simulink model "orbit_propagator_matlab2023b"  (R2023b)
settings: Solver=FixedStepAuto  StartTime=0.0  StopTime=207944  FixedStep=sim_step_size  RelTol=1e-6  AbsTol=1e-7
model workspace (MAT data in the model file):
  current_year = 2025
  year = 2013
values from neighbouring files (symbols this model uses):
  alpha_acc = sqrt(0.7)    [HSat_op_setup_merged_maria.m]    (also in init_orbit_analysis_with_drag_loss.m)
  aph = 200*ones(1,7)    [init_orbit_analysis_with_drag_loss.m]
  COM = [0, 0, 0.25+0.3]    [init_orbit_analysis_with_drag_loss.m]
  ext_ENV_muEarth = 3.986005e14    (= 398600500000000)    [GEO_insertion_setup.m]    (also in HSat_op_setup.m; HSat_op_setup_merged_maria.m; init_orbit_analysis_with_drag_loss.m)
  F107 = 300    [init_orbit_analysis_with_drag_loss.m]
  P_solar = 4.56e-6    (= 4.56e-06)    [HSat_op_setup_merged_maria.m]    (also in init_orbit_analysis_with_drag_loss.m)
  perigee_vector_eci = [0, 1, 0]    [init_orbit_analysis_with_drag_loss.m]
  sim_SC_init_MoI_EOR_wet = [ ... (first row only)    [HSat_op_setup.m]    (also in HSat_op_setup_merged_maria.m; init_orbit_analysis_with_drag_loss.m)
  sim_step_size = 10    [init_orbit_analysis_with_drag_loss.m]
  sun_pointing = 1    [init_orbit_analysis_with_drag_loss.m]
  sun_pointing_SA = 0    [HSat_op_setup_merged_maria.m]    (also in init_orbit_analysis_with_drag_loss.m)
  theta = deg2rad(0)    [init_orbit_analysis_with_drag_loss.m]
undefined symbols (not defined in the file or in its folder): attitude, sun_vector_oc
libraries: aerolibutil x37, matrix_library x37, Toolbox x10, sharedtransform x10, aerolibatmos2 x1, simulink x1, simulink_extras x1
(part 1 of 3)
settings Model: Creator=mariahoflund  LastModifiedBy=mariahoflund
settings OptimizationCC: ReuseModelBlockBuffer=off

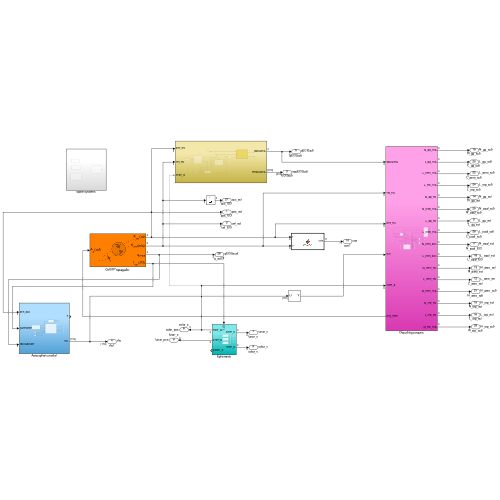
[thumbnail: Simulink's stored preview of the top-level diagram]
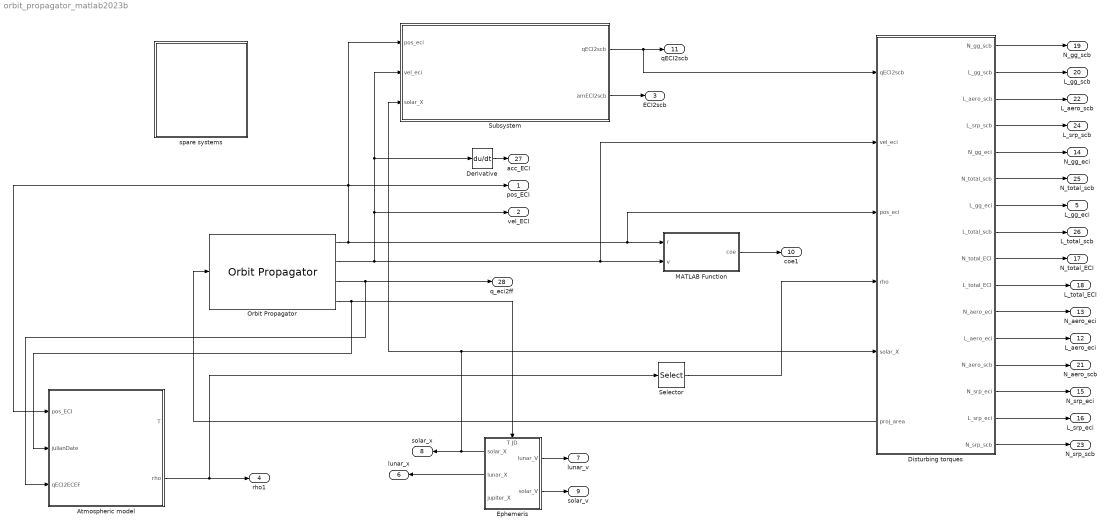
== system orbit_propagator_matlab2023b ==
  Atmospheric model : Subsystem
  Derivative : Derivative
  Disturbing torques : Subsystem
      settings: PortSchema="{\"entries\":[{\"content\":{\"sides\":[{\"content\":{\"connectorIds\":[\"In1\",\"In2\",\"In3\",\"In4\",\"In5\",\"Out17\"]},\"type\":\"ConnectorPlacement.EquallySpacedRectSide\",\"uuid\":\"f7646224-ab06-4eea-96ac-d12bca900cc3\"},{\"content\":{\"connectorIds\":[\"Out1\",\"Out2\",\"Out3\",\"Out4\",\"Out5\",\"Out6\",\"Out7\",\"Out8\",\"Out9\",\"Out10\",\"Out11\",\"Out12\",\"Out13\",\"Out14\",\"Out15\",\"Out16\"],\"side\":\"RIGHT\"},\"type\":\"ConnectorPlacement.EquallySpacedRectSide\",\"uuid\":\"f1692c9b-85c8-425f-b863-5686676bcc52\"},{\"content\":{\"side\":\"TOP\"},\"type\":\"ConnectorPlacement.EquallySpacedRectSide\",\"uuid\":\"99318efc-0d51-43b9-a797-88ad9969849b\"}]},\"type\":\"ConnectorPlacement.EquallySpacedConnector\",\"uuid\":\"1ef90454-3497-43ed-a39d-3078d1204b3e\"}],\"packageUris\":[\"http://schema.mathworks.com/mf0/Connector/R2020b\"],\"version\":\"1.0\"}"
  Ephemeris : Subsystem
      settings: PortSchema="{\"entries\":[{\"content\":{\"sides\":[{\"content\":{\"connectorIds\":[\"Out4\",\"Out5\"]},\"type\":\"ConnectorPlacement.EquallySpacedRectSide\",\"uuid\":\"e633fcf3-0477-4ff0-a81d-4455c68815fb\"},{\"content\":{\"connectorIds\":[\"Out1\",\"Out2\",\"Out3\"],\"side\":\"RIGHT\"},\"type\":\"ConnectorPlacement.EquallySpacedRectSide\",\"uuid\":\"e19e3365-4d80-4524-a5d7-f4214f0f2988\"},{\"content\":{\"connectorIds\":[\"In1\"],\"side\":\"TOP\"},\"type\":\"ConnectorPlacement.EquallySpacedRectSide\",\"uuid\":\"a3adb7cc-79c0-421a-aab6-26119d48c80d\"}]},\"type\":\"ConnectorPlacement.EquallySpacedConnector\",\"uuid\":\"987b98a1-bb11-4f5a-8767-775a43bc92c1\"}],\"packageUris\":[\"http://schema.mathworks.com/mf0/Connector/R2020b\"],\"version\":\"1.0\"}"
  MATLAB Function : MATLAB Function  TreatAsAtomicUnit=on
  Orbit Propagator : OrbitPropagator  propagator=Numerical (high precision)  startDate=2459204.5  mass=mission.Satellite.mass  semiMajorAxis=mission.Satellite.SemiMajorAxis  eccentricity=mission.Satellite.Eccentricity  inclination=mission.Satellite.Inclination  raan=mission.Satellite.RAAN  argPeriapsis=mission.Satellite.ArgOfPeriapsis  trueAnomaly=mission.Satellite.TrueAnomaly  inertialPosition=[3649700.0 3308200.0 -4676600.0]  inertialVelocity=[-2750.8 6666.4 2573.4]  fixedPosition=[-4142689.0 -2676864.7 -4669861.6]  fixedVelocity=[1452.7 -6720.7 2568.1]  customR=3396200  customMu=4.305e13  customJ2=1.0826269e-03  customOmega=4.06125949e-3  shDegree=60  outputTransform=on  useDrag=on  dragCoeff=Cd  dragAreaSrc=Port  dragArea=mission.Satellite.area  includeJupiterGravity=on
  Selector : Selector  InputPortWidth=9  IndexOptions=Index vector (dialog)  Indices=[6]  OutputSizes=1
  Subsystem : Subsystem
  spare systems : Subsystem
  pos_ECI : Outport  SignalName=pos_eci
  vel_ECI : Outport  Port=2  SignalName=vel_eci
  ECI2scb : Outport  Port=3  SignalName=matECI2scb
  rho1 : Outport  Port=4  SignalName=rho
  L_gg_eci : Outport  Port=5  SignalName=L_gg_eci
  lunar_x : Outport  Port=6  SignalName=lunar_pos
  lunar_v : Outport  Port=7  SignalName=lunar_v
  solar_x : Outport  Port=8  SignalName=solar_pos
  solar_v : Outport  Port=9  SignalName=solar_v
  coe1 : Outport  Port=10  SignalName=coe
  qECI2scb : Outport  Port=11  SignalName=qECI2scb
  L_aero_eci : Outport  Port=12  SignalName=L_aero_eci
  N_aero_eci : Outport  Port=13  SignalName=N_aero_eci
  N_gg_eci : Outport  Port=14  SignalName=N_gg_eci
  N_srp_eci : Outport  Port=15  SignalName=N_srp_eci
  L_srp_eci : Outport  Port=16  SignalName=L_srp_eci
  N_total_ECI : Outport  Port=17  SignalName=N_total_eci
  L_total_ECI : Outport  Port=18  SignalName=L_total_eci
  N_gg_scb : Outport  Port=19  SignalName=N_gg_scb
  L_gg_scb : Outport  Port=20  SignalName=L_gg_scb
  N_aero_scb : Outport  Port=21  SignalName=N_aero_scb
  L_aero_scb : Outport  Port=22  SignalName=L_aero_scb
  N_srp_scb : Outport  Port=23  SignalName=N_srp_scb
  L_srp_scb : Outport  Port=24  SignalName=L_srp_scb
  N_total_scb : Outport  Port=25  SignalName=N_total_scb
  L_total_scb : Outport  Port=26  SignalName=L_total_scb
  acc_ECI : Outport  Port=27  SignalName=acc_eci
  q_eci2ff : Outport  Port=28  SignalName=qECI2ecef
  wires:
  Ephemeris/2(lunar_X) -> lunar_x/1
  Orbit Propagator/4 -> Ephemeris/1(T JD), Atmospheric model/2(julianDate)
  MATLAB Function/1(coe) -> coe1/1
  Orbit Propagator/2 -> Subsystem/2(vel_eci), Derivative/1, vel_ECI/1, Disturbing torques/2(vel_eci), MATLAB Function/2(v)
  Ephemeris/4(lunar_V) -> lunar_v/1
  Ephemeris/5(solar_V) -> solar_v/1
  Orbit Propagator/1 -> Atmospheric model/1(pos_ECI), Subsystem/1(pos_eci), pos_ECI/1, MATLAB Function/1(r), Disturbing torques/3(pos_eci)
  Derivative/1 -> acc_ECI/1
  Orbit Propagator/3 -> q_eci2ff/1, Atmospheric model/3(qECI2ECEF)
  Ephemeris/1(solar_X) -> Subsystem/3(solar_X), Disturbing torques/5(solar_X), solar_x/1
  Selector/1 -> Disturbing torques/4(rho)
  Disturbing torques/1(N_gg_scb) -> N_gg_scb/1
  Disturbing torques/2(L_gg_scb) -> L_gg_scb/1
  Disturbing torques/3(L_aero_scb) -> L_aero_scb/1
  Disturbing torques/4(L_srp_scb) -> L_srp_scb/1
  Disturbing torques/5(N_gg_eci) -> N_gg_eci/1
  Disturbing torques/6(N_total_scb) -> N_total_scb/1
  Disturbing torques/7(L_gg_eci) -> L_gg_eci/1
  Disturbing torques/8(L_total_scb) -> L_total_scb/1
  Disturbing torques/9(N_total_ECI) -> N_total_ECI/1
  Disturbing torques/17(proj_area) -> Orbit Propagator/1
  Disturbing torques/10(L_total_ECI) -> L_total_ECI/1
  Disturbing torques/11(N_aero_eci) -> N_aero_eci/1
  Disturbing torques/12(L_aero_eci) -> L_aero_eci/1
  Disturbing torques/13(N_aero_scb) -> N_aero_scb/1
  Disturbing torques/14(N_srp_eci) -> N_srp_eci/1
  Disturbing torques/15(L_srp_eci) -> L_srp_eci/1
  Disturbing torques/16(N_srp_scb) -> N_srp_scb/1
  Atmospheric model/2(rho) -> rho1/1, Selector/1
  Subsystem/1(qECI2scb) -> Disturbing torques/1(qECI2scb), qECI2scb/1
  Subsystem/2(amECI2scb) -> ECI2scb/1

== system orbit_propagator_matlab2023b/Atmospheric model ==
  pos_ECI : Inport
  julianDate : Inport  Port=2
  qECI2ECEF : Inport  Port=3
  F107 : Constant  Value=F107
  F107a : Constant  Value=F107
  MATLAB Function1 : MATLAB Function  TreatAsAtomicUnit=on
  NRLMSISE-00 Atmosphere Model : aerolibatmos2/NRLMSISE-00 Atmosphere Model  units=Metric (MKS)  lst_input=off  flux_ap_input=on  flags_input=Internal  flags=ones(1,23)  oxygen_in=off  action=Warning
  aph : Constant  Value=aph
  pos_eci to lla : Subsystem
  T : Outport
  rho : Outport  Port=2
  wires:
  NRLMSISE-00 Atmosphere Model/2 -> rho/1
  qECI2ECEF/1 -> pos_eci to lla/2(qECI2ECEF)
  julianDate/1 -> MATLAB Function1/1(julianDate)
  F107/1 -> NRLMSISE-00 Atmosphere Model/6
  NRLMSISE-00 Atmosphere Model/1 -> T/1
  MATLAB Function1/1(yr) -> NRLMSISE-00 Atmosphere Model/2
  pos_ECI/1 -> pos_eci to lla/1(pos_ECI)
  aph/1 -> NRLMSISE-00 Atmosphere Model/7
  MATLAB Function1/2(dayOfYear) -> NRLMSISE-00 Atmosphere Model/3
  pos_eci to lla/1(Out1) -> NRLMSISE-00 Atmosphere Model/1  "lat,long,alt"
  F107a/1 -> NRLMSISE-00 Atmosphere Model/5
  MATLAB Function1/3(timeUTSeconds) -> NRLMSISE-00 Atmosphere Model/4

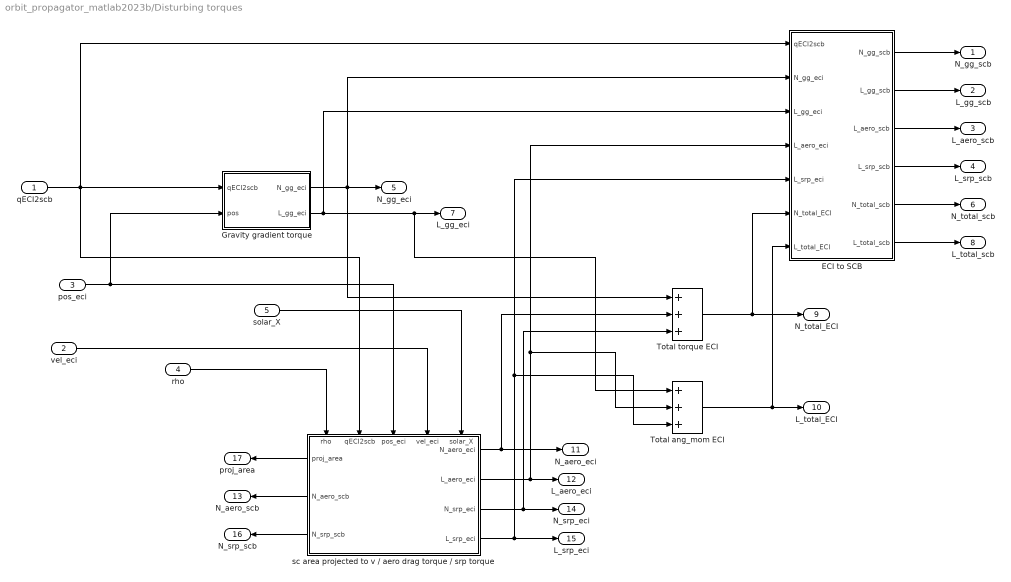
== system orbit_propagator_matlab2023b/Disturbing torques ==
  qECI2scb : Inport
  vel_eci : Inport  Port=2
  pos_eci : Inport  Port=3
  rho : Inport  Port=4
  solar_X : Inport  Port=5
  ECI to SCB : Subsystem
  Gravity gradient torque : Subsystem
  Total ang_mom ECI : Sum  Inputs=+++
  Total torque ECI : Sum  Inputs=+++
  sc area projected to v / aero drag torque / srp torque : Subsystem
      settings: PortSchema="{\"entries\":[{\"content\":{\"sides\":[{\"content\":{\"connectorIds\":[\"Out5\",\"Out6\",\"Out7\"]},\"type\":\"ConnectorPlacement.EquallySpacedRectSide\",\"uuid\":\"2286bbd5-74fd-4e7a-af53-1dba63e33399\"},{\"content\":{\"connectorIds\":[\"Out1\",\"Out2\",\"Out3\",\"Out4\"],\"side\":\"RIGHT\"},\"type\":\"ConnectorPlacement.EquallySpacedRectSide\",\"uuid\":\"14ee861f-d330-4e3d-9d37-eadf89803ba2\"},{\"content\":{\"connectorIds\":[\"In1\",\"In2\",\"In3\",\"In4\",\"In5\"],\"side\":\"TOP\"},\"type\":\"ConnectorPlacement.EquallySpacedRectSide\",\"uuid\":\"a82f7821-7262-41d9-9ef8-416bfb7d6f77\"}]},\"type\":\"ConnectorPlacement.EquallySpacedConnector\",\"uuid\":\"26570817-76bd-4bb8-9b49-7b0dee7f17a2\"}],\"packageUris\":[\"http://schema.mathworks.com/mf0/Connector/R2020b\"],\"version\":\"1.0\"}"
  N_gg_scb : Outport
  L_gg_scb : Outport  Port=2
  L_aero_scb : Outport  Port=3
  L_srp_scb : Outport  Port=4
  N_gg_eci : Outport  Port=5
  N_total_scb : Outport  Port=6
  L_gg_eci : Outport  Port=7
  L_total_scb : Outport  Port=8
  N_total_ECI : Outport  Port=9
  L_total_ECI : Outport  Port=10
  N_aero_eci : Outport  Port=11
  L_aero_eci : Outport  Port=12
  N_aero_scb : Outport  Port=13
  N_srp_eci : Outport  Port=14
  L_srp_eci : Outport  Port=15
  N_srp_scb : Outport  Port=16
  proj_area : Outport  Port=17
  wires:
  pos_eci/1 -> Gravity gradient torque/2(pos), sc area projected to v / aero drag torque / srp torque/3(pos_eci)
  sc area projected to v / aero drag torque / srp torque/5(proj_area) -> proj_area/1
  Gravity gradient torque/2(L_gg_eci) -> L_gg_eci/1, Total ang_mom ECI/1, ECI to SCB/3(L_gg_eci)
  sc area projected to v / aero drag torque / srp torque/4(L_srp_eci) -> ECI to SCB/5(L_srp_eci), Total ang_mom ECI/3, L_srp_eci/1
  rho/1 -> sc area projected to v / aero drag torque / srp torque/1(rho)
  ECI to SCB/4(L_srp_scb) -> L_srp_scb/1
  ECI to SCB/5(N_total_scb) -> N_total_scb/1
  solar_X/1 -> sc area projected to v / aero drag torque / srp torque/5(solar_X)
  ECI to SCB/3(L_aero_scb) -> L_aero_scb/1
  sc area projected to v / aero drag torque / srp torque/3(N_srp_eci) -> Total torque ECI/3, N_srp_eci/1
  Total torque ECI/1 -> ECI to SCB/6(N_total_ECI), N_total_ECI/1
  ECI to SCB/6(L_total_scb) -> L_total_scb/1
  ECI to SCB/2(L_gg_scb) -> L_gg_scb/1
  sc area projected to v / aero drag torque / srp torque/1(N_aero_eci) -> Total torque ECI/2, N_aero_eci/1
  ECI to SCB/1(N_gg_scb) -> N_gg_scb/1
  Total ang_mom ECI/1 -> ECI to SCB/7(L_total_ECI), L_total_ECI/1
  qECI2scb/1 -> ECI to SCB/1(qECI2scb), sc area projected to v / aero drag torque / srp torque/2(qECI2scb), Gravity gradient torque/1(qECI2scb)
  sc area projected to v / aero drag torque / srp torque/7(N_srp_scb) -> N_srp_scb/1
  Gravity gradient torque/1(N_gg_eci) -> Total torque ECI/1, N_gg_eci/1, ECI to SCB/2(N_gg_eci)
  sc area projected to v / aero drag torque / srp torque/6(N_aero_scb) -> N_aero_scb/1
  vel_eci/1 -> sc area projected to v / aero drag torque / srp torque/4(vel_eci)
  sc area projected to v / aero drag torque / srp torque/2(L_aero_eci) -> ECI to SCB/4(L_aero_eci), Total ang_mom ECI/2, L_aero_eci/1

== system orbit_propagator_matlab2023b/Ephemeris ==
  T JD : Inport
  Gain{,1..3} (4 alike) : Gain  Gain=1000
  Jupiter Ephemeris : PlanetaryEphem  target=Jupiter
  Lunar Ephemeris : PlanetaryEphem
  Solar Ephemeris : PlanetaryEphem  target=Sun
  km to m : Gain  Gain=1000
  km to m1 : Gain  Gain=1000
  solar_X : Outport
  lunar_X : Outport  Port=2
  jupiter_X : Outport  Port=3
  lunar_V : Outport  Port=4
  solar_V : Outport  Port=5
  wires:
  T JD/1 -> Lunar Ephemeris/1, Jupiter Ephemeris/1, Solar Ephemeris/1
  Lunar Ephemeris/2 -> Gain1/1
  Solar Ephemeris/1 -> Gain2/1
  Solar Ephemeris/2 -> km to m/1
  Lunar Ephemeris/1 -> Gain/1
  Gain/1 -> lunar_X/1
  Gain1/1 -> lunar_V/1
  Gain2/1 -> solar_X/1
  km to m/1 -> solar_V/1
  Jupiter Ephemeris/2 -> km to m1/1
  Gain3/1 -> jupiter_X/1
  km to m1/1 -> ?
  Jupiter Ephemeris/1 -> Gain3/1

== system orbit_propagator_matlab2023b/Subsystem ==
  pos_eci : Inport
  vel_eci : Inport  Port=2
  solar_X : Inport  Port=3
  Attitude : Subsystem  Variant=on  VariantControlMode=label  VariantControl=Choice  LabelModeActiveChoice=nadir  PropagateVariantConditions=on
  Constant : Constant  Value=sun_pointing
  Merge : Merge
  Switch Case : SwitchCase
  sun pointing in orbit plane : Subsystem  TreatAsAtomicUnit=on
  sun pointing out of plane : Subsystem  TreatAsAtomicUnit=on
  qECI2scb : Outport
  amECI2scb : Outport  Port=2
  wires:
  Attitude/1(qECI2scb) -> qECI2scb/1
  vel_eci/1 -> sun pointing in orbit plane/2(vel_eci), Attitude/2(velECI)
  Attitude/2(amECI2scb) -> amECI2scb/1
  pos_eci/1 -> sun pointing in orbit plane/3(pos_eci), Attitude/1(posECI)
  Switch Case/2 -> sun pointing out of plane/Action
  Switch Case/1 -> sun pointing in orbit plane/Action
  solar_X/1 -> sun pointing in orbit plane/1(solar_X), sun pointing out of plane/1(solar_X)
  sun pointing in orbit plane/1(Out1) -> Merge/1
  sun pointing out of plane/1(Out1) -> Merge/2
  Merge/1 -> Attitude/3(solar_X)
  Constant/1 -> Switch Case/1

== system orbit_propagator_matlab2023b/spare systems ==
  LST calculation : Subsystem  Commented=on
  Subsystem : Subsystem  Commented=on
  create custom sun vector : Subsystem  Commented=on
      settings: PortSchema="{\"entries\":[{\"content\":{\"sides\":[{\"content\":{},\"type\":\"ConnectorPlacement.EquallySpacedRectSide\",\"uuid\":\"5755fe33-27e5-4fac-b1a9-828212356ffb\"},{\"content\":{\"connectorIds\":[\"Out1\"],\"side\":\"RIGHT\"},\"type\":\"ConnectorPlacement.EquallySpacedRectSide\",\"uuid\":\"342e2dfb-ebd3-43c9-8218-dffda7908936\"},{\"content\":{\"connectorIds\":[\"In1\",\"In2\"],\"side\":\"TOP\"},\"type\":\"ConnectorPlacement.EquallySpacedRectSide\",\"uuid\":\"c86662bf-fbb1-4b53-aebd-7f62bd217376\"}]},\"type\":\"ConnectorPlacement.EquallySpacedConnector\",\"uuid\":\"2e470c5a-53cc-4a23-914f-bd86fdc85ade\"}],\"packageUris\":[\"http://schema.mathworks.com/mf0/Connector/R2020b\"],\"version\":\"1.0\"}"
  sun_angle_slo : Subsystem  Commented=on
      settings: PortSchema="{\"entries\":[{\"content\":{\"sides\":[{\"content\":{\"connectorIds\":[\"In1\",\"In2\"]},\"type\":\"ConnectorPlacement.EquallySpacedRectSide\",\"uuid\":\"2286bbd5-74fd-4e7a-af53-1dba63e33399\"},{\"content\":{\"side\":\"RIGHT\"},\"type\":\"ConnectorPlacement.EquallySpacedRectSide\",\"uuid\":\"14ee861f-d330-4e3d-9d37-eadf89803ba2\"},{\"content\":{\"side\":\"TOP\"},\"type\":\"ConnectorPlacement.EquallySpacedRectSide\",\"uuid\":\"a82f7821-7262-41d9-9ef8-416bfb7d6f77\"},{\"content\":{\"connectorIds\":[\"Out1\"],\"side\":\"BOTTOM\"},\"type\":\"ConnectorPlacement.EquallySpacedRectSide\",\"uuid\":\"582a2bf6-c053-407d-b600-dfbf3f97abd6\"}]},\"type\":\"ConnectorPlacement.EquallySpacedConnector\",\"uuid\":\"26570817-76bd-4bb8-9b49-7b0dee7f17a2\"}],\"packageUris\":[\"http://schema.mathworks.com/mf0/Connector/R2020b\"],\"version\":\"1.0\"}"

== system orbit_propagator_matlab2023b/Atmospheric model/pos_eci to lla ==
  pos_ECI : Inport
  qECI2ECEF : Inport  Port=2
  ECEF Position to LLA : ECEF2LLA
  Mux : Mux  Inputs=2
  Quaternion Rotation : aerolibutil/Quaternion Rotation
  Out1 : Outport
  wires:
  pos_ECI/1 -> Quaternion Rotation/2
  qECI2ECEF/1 -> Quaternion Rotation/1
  Quaternion Rotation/1 -> ECEF Position to LLA/1
  ECEF Position to LLA/1 -> Mux/1
  ECEF Position to LLA/2 -> Mux/2
  Mux/1 -> Out1/1

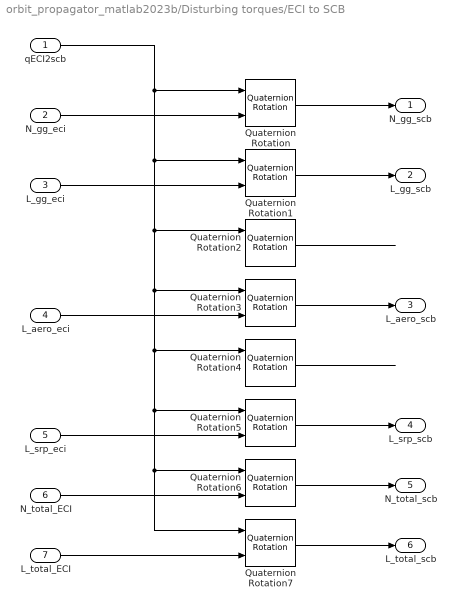
== system orbit_propagator_matlab2023b/Disturbing torques/ECI to SCB ==
  qECI2scb : Inport
  N_gg_eci : Inport  Port=2
  L_gg_eci : Inport  Port=3
  L_aero_eci : Inport  Port=4
  L_srp_eci : Inport  Port=5
  N_total_ECI : Inport  Port=6
  L_total_ECI : Inport  Port=7
  Quaternion Rotation{,1..7} (8 alike) : aerolibutil/Quaternion Rotation
  N_gg_scb : Outport
  L_gg_scb : Outport  Port=2
  L_aero_scb : Outport  Port=3
  L_srp_scb : Outport  Port=4
  N_total_scb : Outport  Port=5
  L_total_scb : Outport  Port=6
  wires:
  qECI2scb/1 -> Quaternion Rotation1/1, Quaternion Rotation2/1, Quaternion Rotation3/1, Quaternion Rotation4/1, Quaternion Rotation7/1, Quaternion Rotation6/1, Quaternion Rotation5/1, Quaternion Rotation/1
  N_gg_eci/1 -> Quaternion Rotation/2
  Quaternion Rotation/1 -> N_gg_scb/1
  Quaternion Rotation1/1 -> L_gg_scb/1
  L_gg_eci/1 -> Quaternion Rotation1/2
  Quaternion Rotation2/1 -> ?
  ? -> Quaternion Rotation2/2
  Quaternion Rotation3/1 -> L_aero_scb/1
  L_aero_eci/1 -> Quaternion Rotation3/2
  Quaternion Rotation4/1 -> ?
  ? -> Quaternion Rotation4/2
  Quaternion Rotation5/1 -> L_srp_scb/1
  L_srp_eci/1 -> Quaternion Rotation5/2
  Quaternion Rotation6/1 -> N_total_scb/1
  Quaternion Rotation7/1 -> L_total_scb/1
  L_total_ECI/1 -> Quaternion Rotation7/2
  N_total_ECI/1 -> Quaternion Rotation6/2

== system orbit_propagator_matlab2023b/Disturbing torques/Gravity gradient torque ==
  qECI2scb : Inport
  pos : Inport  Port=2
  Constant4 : Constant  Value=sim_SC_init_MoI_EOR_wet
  Constant5 : Constant  Value=-5
  Constant6 : Constant  Value=3
  Constant7 : Constant  Value=ext_ENV_muEarth
  Cross Product1 : matrix_library/Cross Product
  Dot Product1 : DotProduct  OutDataTypeStr=Inherit: Inherit via internal rule
  Integrator : Integrator
  Math Function1 : Math  Operator=pow
  Product1 : Product  Inputs=4
  Product2 : Product  Multiplication=Matrix(*)
  Quaternion Inverse : aerolibutil/Quaternion Inverse
  Quaternion Rotation : aerolibutil/Quaternion Rotation
  Quaternion Rotation1 : aerolibutil/Quaternion Rotation
  Sqrt1 : Sqrt
  N_gg_eci : Outport
  L_gg_eci : Outport  Port=2
  wires:
  Constant5/1 -> Math Function1/2
  Sqrt1/1 -> Math Function1/1
  pos/1 -> Quaternion Rotation1/2, Dot Product1/1, Dot Product1/2, Cross Product1/1
  Constant6/1 -> Product1/3
  Math Function1/1 -> Product1/2
  Product1/1 -> Cross Product1/2
  Dot Product1/1 -> Sqrt1/1
  Constant7/1 -> Product1/4
  qECI2scb/1 -> Quaternion Rotation1/1, Quaternion Inverse/1
  Quaternion Inverse/1 -> Quaternion Rotation/1
  Quaternion Rotation/1 -> Product1/1
  Quaternion Rotation1/1 -> Product2/2  "pos_scb"
  Constant4/1 -> Product2/1
  Product2/1 -> Quaternion Rotation/2
  Cross Product1/1 -> Integrator/1, N_gg_eci/1
  Integrator/1 -> L_gg_eci/1

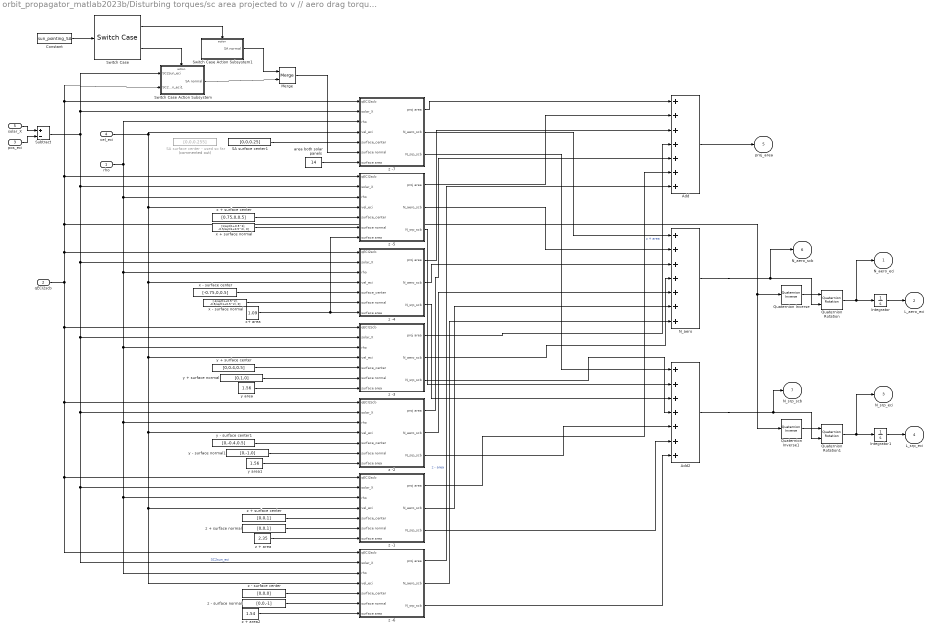
== system orbit_propagator_matlab2023b/Disturbing torques/sc area projected to v // aero drag torque // srp torque ==
  rho : Inport
  qECI2scb : Inport  Port=2
  pos_eci : Inport  Port=3
  vel_eci : Inport  Port=4
  solar_X : Inport  Port=5
  Add : Sum  Inputs=+++++++
  Add2 : Sum  Inputs=+++++++
  Constant : Constant  Value=sun_pointing_SA
  Integrator : Integrator
  Integrator1 : Integrator
  Merge : Merge
  N_aero : Sum  Inputs=+++++++
  Quaternion Inverse : aerolibutil/Quaternion Inverse
  Quaternion Inverse1 : aerolibutil/Quaternion Inverse
  Quaternion Rotation : aerolibutil/Quaternion Rotation
  Quaternion Rotation1 : aerolibutil/Quaternion Rotation
  SA surface center - used so far : Constant  Commented=on  Value=[0,0,0.255]
  SA surface center1 : Constant  Value=[0,0,0.25]
  Subtract : Sum  Inputs=+-
  Switch Case : SwitchCase
  Switch Case Action Subsystem : Subsystem  TreatAsAtomicUnit=on
  Switch Case Action Subsystem1 : Subsystem  TreatAsAtomicUnit=on
  area both solar panels : Constant  Value=14
  x + surface center : Constant  Value=[0.75,0,0.5]
  x + surface normal : Constant  Value=[1/sqrt(1+0.5^2), -0.5/sqrt(1+0.5^2), 0]
  x - surface center : Constant  Value=[-0.75,0,0.5]
  x - surface normal : Constant  Value=[-1/sqrt(1+0.5^2), -0.5/sqrt(1+0.5^2), 0]
  x+ area : Constant  Value=1.09
  y + surface center : Constant  Value=[0,0.4,0.5]
  y + surface normal : Constant  Value=[0,1,0]
  y - surface center1 : Constant  Value=[0,-0.4,0.5]
  y - surface normal1 : Constant  Value=[0,-1,0]
  y area : Constant  Value=1.56
  y area1 : Constant  Value=1.56
  z + area : Constant  Value=2.35
  z + area2 : Constant  Value=1.54
  z + surface center : Constant  Value=[0,0,1]
  z + surface normal : Constant  Value=[0,0,1]
  z - surface center : Constant  Value=[0,0,0]
  z - surface normal : Constant  Value=[0,0,-1]
  z -1 : Subsystem
  z -2 : Subsystem
  z -3 : Subsystem
  z -4 : Subsystem
  z -5 : Subsystem
  z -6 : Subsystem
  z -7 : Subsystem
  N_aero_eci : Outport
  L_aero_eci : Outport  Port=2
  N_srp_eci : Outport  Port=3
  L_srp_eci : Outport  Port=4
  proj_area : Outport  Port=5
  N_aero_scb : Outport  Port=6
  N_srp_scb : Outport  Port=7
  wires:
  z -1/1(proj area) -> Add/6  "z + area"
  Add/1 -> proj_area/1
  area both solar panels/1 -> z -7/7(surface area)
  Subtract/1 -> Switch Case Action Subsystem/1(SC2sun_eci), z -7/2(solar_X), z -5/2(solar_X), z -4/2(solar_X), z -3/2(solar_X), z -2/2(solar_X), z -6/2(solar_X), z -1/2(solar_X)  "SC2sun_eci"
  z -6/1(proj area) -> Add/7  "z - area"
  z - surface normal/1 -> z -6/6(surface normal)
  z + area2/1 -> z -6/7(surface area)
  z - surface center/1 -> z -6/5(surface_center)
  z + surface normal/1 -> z -1/6(surface normal)
  z + area/1 -> z -1/7(surface area)
  z + surface center/1 -> z -1/5(surface_center)
  y + surface normal/1 -> z -3/6(surface normal)
  y area/1 -> z -3/7(surface area)
  y + surface center/1 -> z -3/5(surface_center)
  y - surface normal1/1 -> z -2/6(surface normal)
  y - surface center1/1 -> z -2/5(surface_center)
  rho/1 -> z -7/3(rho), z -5/3(rho), z -4/3(rho), z -3/3(rho), z -2/3(rho), z -6/3(rho), z -1/3(rho)
  y area1/1 -> z -2/7(surface area)
  z -2/1(proj area) -> Add/5
  vel_eci/1 -> z -5/4(vel_eci), z -4/4(vel_eci), z -3/4(vel_eci), z -2/4(vel_eci), z -6/4(vel_eci), z -1/4(vel_eci), z -7/4(vel_eci)
  z -3/1(proj area) -> Add/4
  x - surface normal/1 -> z -4/6(surface normal)
  x - surface center/1 -> z -4/5(surface_center)
  x+ area/1 -> z -4/7(surface area), z -5/7(surface area)
  x + surface normal/1 -> z -5/6(surface normal)
  x + surface center/1 -> z -5/5(surface_center)
  z -4/1(proj area) -> Add/3
  z -5/1(proj area) -> Add/2
  z -5/2(N_aero_scb) -> N_aero/2
  z -4/2(N_aero_scb) -> N_aero/3
  z -3/2(N_aero_scb) -> N_aero/4
  z -2/2(N_aero_scb) -> N_aero/5
  z -1/2(N_aero_scb) -> N_aero/6
  z -6/2(N_aero_scb) -> N_aero/7
  SA surface center1/1 -> z -7/5(surface_center)
  z -7/1(proj area) -> Add/1
  z -7/2(N_aero_scb) -> N_aero/1
  N_aero/1 -> N_aero_scb/1, Quaternion Rotation/2
  Quaternion Rotation/1 -> N_aero_eci/1, Integrator/1
  Integrator/1 -> L_aero_eci/1
  Quaternion Inverse/1 -> Quaternion Rotation/1
  Add2/1 -> N_srp_scb/1, Quaternion Rotation1/2
  Quaternion Inverse1/1 -> Quaternion Rotation1/1
  Quaternion Rotation1/1 -> N_srp_eci/1, Integrator1/1
  qECI2scb/1 -> z -3/1(qECI2scb), z -2/1(qECI2scb), z -6/1(qECI2scb), z -1/1(qECI2scb), z -4/1(qECI2scb), Switch Case Action Subsystem/2(SC2sun_eci1), z -7/1(qECI2scb), z -5/1(qECI2scb), Quaternion Inverse1/1, Quaternion Inverse/1
  Integrator1/1 -> L_srp_eci/1
  z -7/3(N_srp_scb) -> Add2/1
  z -5/3(N_srp_scb) -> Add2/2
  z -4/3(N_srp_scb) -> Add2/3
  z -3/3(N_srp_scb) -> Add2/4
  z -2/3(N_srp_scb) -> Add2/5
  z -1/3(N_srp_scb) -> Add2/6
  z -6/3(N_srp_scb) -> Add2/7
  solar_X/1 -> Subtract/1
  pos_eci/1 -> Subtract/2
  Switch Case Action Subsystem/1(SA normal) -> Merge/2
  Switch Case/2 -> Switch Case Action Subsystem/Action
  Switch Case/1 -> Switch Case Action Subsystem1/Action
  Switch Case Action Subsystem1/1(SA normal) -> Merge/1
  Merge/1 -> z -7/6(surface normal)
  Constant/1 -> Switch Case/1

== system orbit_propagator_matlab2023b/Subsystem/Attitude ==
  posECI : Inport
  velECI : Inport  Port=2
  solar_X : Inport  Port=3
  Att z towards the sun : Subsystem  VariantControl=z_sun
  Att z towards the sun and rotation around z : Subsystem  VariantControl=z_sun_rot
  att: z in v : Subsystem  VariantControl=z_in_v
  changes with altitude : Subsystem  VariantControl=varying
  q (z in r) : Subsystem  VariantControl=nadir
  qECI2scb : Outport
  amECI2scb : Outport  Port=2

== system orbit_propagator_matlab2023b/Subsystem/sun pointing in orbit plane ==
  solar_X : Inport
  vel_eci : Inport  Port=2
  pos_eci : Inport  Port=3
  Action Port : ActionPort  ActionPortLabel=case [ 1 ]:
  Cross Product : matrix_library/Cross Product
  Cross Product1 : matrix_library/Cross Product
  Cross Product2 : matrix_library/Cross Product
  Nomalize_noDivideByZero1 : Subsystem
      mask Display: disp('u/||u||')
  Nomalize_noDivideByZero3 : Subsystem
      mask Display: disp('u/||u||')
  Out1 : Outport
  wires:
  solar_X/1 -> Cross Product1/2
  Nomalize_noDivideByZero1/1(ehat) -> Cross Product/1
  vel_eci/1 -> Nomalize_noDivideByZero3/1(e)
  Cross Product2/1 -> Out1/1  "orbit tangent in sun direction"
  Cross Product1/1 -> Cross Product2/1  "orbit tangent"
  pos_eci/1 -> Nomalize_noDivideByZero1/1(e)
  Cross Product/1 -> Cross Product2/2, Cross Product1/1  "orbit normal"
  Nomalize_noDivideByZero3/1(ehat) -> Cross Product/2

== system orbit_propagator_matlab2023b/Subsystem/sun pointing out of plane ==
  solar_X : Inport
  Action Port : ActionPort  ActionPortLabel=default:
  Out1 : Outport
  wires:
  solar_X/1 -> Out1/1

== system orbit_propagator_matlab2023b/spare systems/LST calculation ==
  UT : Inport
  mu : Inport  Port=2
  Add : Sum
  Constant : Constant  Value=3600
  Constant1 : Constant  Value=15
  Divide : Product  Inputs=*/
  Divide1 : Product  Inputs=*/
  Extarct longitude : matrix_library/Submatrix  RowSpan=One row  RowStartMode=Index  RowStartIndex=2  RowEndMode=Last  RowEndIndex=1  ColSpan=All columns  ColStartMode=Index  ColStartIndex=2  ColEndMode=Last  ColEndIndex=1
  LST : Outport
  wires:
  UT/1 -> Divide/1
  Constant/1 -> Divide/2
  mu/1 -> Extarct longitude/1
  Extarct longitude/1 -> Divide1/1
  Constant1/1 -> Divide1/2
  Add/1 -> LST/1
  Divide/1 -> Add/2
  Divide1/1 -> Add/1

== system orbit_propagator_matlab2023b/spare systems/Subsystem ==
  pos_eci : Inport
  qeci2ff : Inport  Port=2
  "Long, Lat" : Constant  Value=[67, 20]
  Quaternion Rotation : aerolibutil/Quaternion Rotation
  angle : Constant  Value=80
  within sight : Subsystem
  within sight boolean : Outport
  wires:
  qeci2ff/1 -> Quaternion Rotation/1
  pos_eci/1 -> Quaternion Rotation/2
  Quaternion Rotation/1 -> within sight/1(pos_ecef)
  "Long, Lat"/1 -> within sight/2("GS long, lat (deg)")
  angle/1 -> within sight/3(view angle)
  within sight/1(within sight boolean) -> within sight boolean/1

== system orbit_propagator_matlab2023b/spare systems/create custom sun vector ==
  vel_eci : Inport
  pos_eci : Inport  Port=2
  Constant1 : Constant  Value=sun_vector_oc
  Constant2 : Constant  Value=perigee_vector_eci
  Cross Product : matrix_library/Cross Product
  Cross Product1 : matrix_library/Cross Product
  Direction Cosine Matrix to Quaternions : sharedtransform/Direction Cosine Matrix  to Quaternions  aMode=0  action=None  tolerance=eps(2)
      settings: LibrarySourceBlock=|
      | aerolibtransform2/Direction Cosine Matrix
      | to Quaternions
  Matrix Concatenate : Concatenate  NumInputs=3  Mode=Multidimensional array
  Nomalize_noDivideByZero1 : Subsystem
      mask Display: disp('u/||u||')
  Nomalize_noDivideByZero2 : Subsystem
      mask Display: disp('u/||u||')
  Quaternion Inverse : aerolibutil/Quaternion Inverse
  Quaternion Rotation2 : aerolibutil/Quaternion Rotation
  x : Reshape  OutputDimensionality=Row vector (2-D)
  y : Reshape  OutputDimensionality=Row vector (2-D)
  z : Reshape  OutputDimensionality=Row vector (2-D)
  sun_vector_eci : Outport
  wires:
  vel_eci/1 -> Cross Product/2
  pos_eci/1 -> Cross Product/1
  Cross Product/1 -> Nomalize_noDivideByZero1/1(e)  "orbit normal"
  Constant2/1 -> Nomalize_noDivideByZero2/1(e)
  Nomalize_noDivideByZero2/1(ehat) -> Cross Product1/2, x/1
  z/1 -> Matrix Concatenate/3
  y/1 -> Matrix Concatenate/2
  x/1 -> Matrix Concatenate/1
  Matrix Concatenate/1 -> Direction Cosine Matrix to Quaternions/1
  Cross Product1/1 -> y/1
  Direction Cosine Matrix to Quaternions/1 -> Quaternion Inverse/1  "ECI2robit"
  Constant1/1 -> Quaternion Rotation2/2  "sun_vector_obrit_coord"
  Nomalize_noDivideByZero1/1(ehat) -> z/1, Cross Product1/1
  Quaternion Inverse/1 -> Quaternion Rotation2/1
  Quaternion Rotation2/1 -> sun_vector_eci/1  "sun_vector_eci"

== system orbit_propagator_matlab2023b/spare systems/sun_angle_slo ==
  q_ECI2slo : Inport
  sun_pos_eci : Inport  Port=2
  Acos : Trigonometry  Operator=acos
  Constant : Constant  Value=[1,0,1]
  Constant1 : Constant  Value=[0,0,1]
  Dot Product : DotProduct  OutDataTypeStr=Inherit: Inherit via internal rule
  Nomalize_noDivideByZero : Subsystem
      mask Display: disp('u/||u||')
  Quaternion Rotation : aerolibutil/Quaternion Rotation
  element-wise multiplication : Product
  sun_angle_slo : Outport
  wires:
  q_ECI2slo/1 -> Quaternion Rotation/1
  sun_pos_eci/1 -> Quaternion Rotation/2
  Quaternion Rotation/1 -> element-wise multiplication/1  "sun_pos_slo"
  Constant/1 -> element-wise multiplication/2
  element-wise multiplication/1 -> Nomalize_noDivideByZero/1(e)
  Constant1/1 -> Dot Product/2
  Nomalize_noDivideByZero/1(ehat) -> Dot Product/1
  Dot Product/1 -> Acos/1
  Acos/1 -> sun_angle_slo/1

== system orbit_propagator_matlab2023b/Disturbing torques/sc area projected to v // aero drag torque // srp torque/Switch Case Action Subsystem ==
  SC2sun_eci : Inport
  SC2sun_eci1 : Inport  Port=2
  Action Port : ActionPort  ActionPortLabel=default:
  Constant : Constant  Value=[1, 0, 1]
  Product : Product
  sun pointing solar arrays : Subsystem
  SA normal : Outport
  wires:
  SC2sun_eci/1 -> sun pointing solar arrays/1(SC2sun_eci)
  SC2sun_eci1/1 -> sun pointing solar arrays/2(qECI2scb)
  sun pointing solar arrays/1(SA normal) -> Product/1
  Constant/1 -> Product/2
  Product/1 -> SA normal/1

== system orbit_propagator_matlab2023b/Disturbing torques/sc area projected to v // aero drag torque // srp torque/Switch Case Action Subsystem1 ==
  Action Port : ActionPort  ActionPortLabel=case [ 1 ]:
  Constant : Constant  Value=[0, 0, 1]
  SA normal : Outport
  wires:
  Constant/1 -> SA normal/1

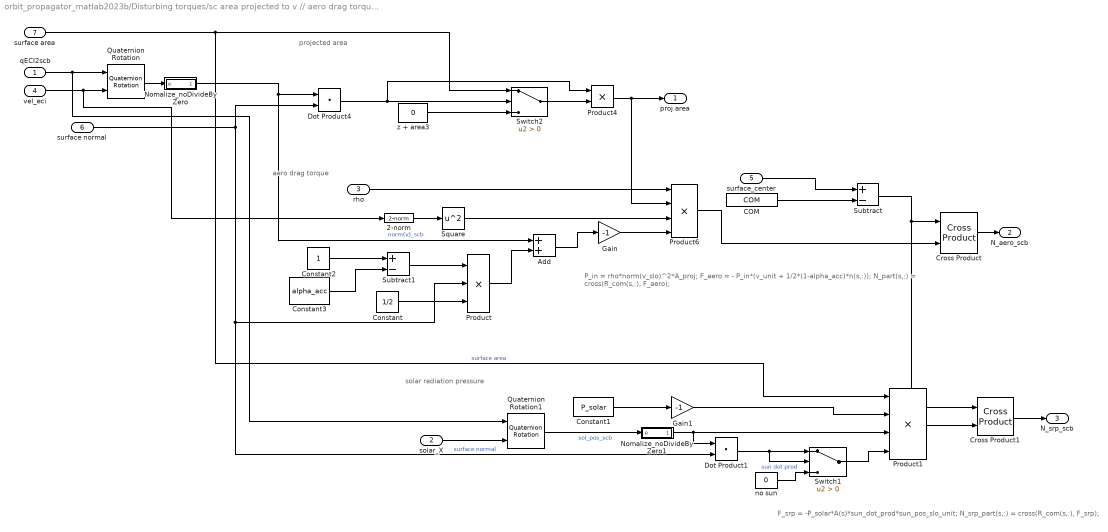
== system orbit_propagator_matlab2023b/Disturbing torques/sc area projected to v // aero drag torque // srp torque/z -1 ==
  note: projected area
  note: aero drag torque
  note: solar radiation pressure
  note: P_in = rho*norm(v_slo)^2*A_proj;
      | F_aero = - P_in*(v_unit + 1/2*(1-alpha_acc)*n(s,:));
      | N_part(s,:) = cross(R_com(s,:), F_aero);
  note: F_srp = -P_solar*A(s)*sun_dot_prod*sun_pos_slo_unit;
      | N_srp_part(s,:) = cross(R_com(s,:), F_srp);
  qECI2scb : Inport
  solar_X : Inport  Port=2
  rho : Inport  Port=3
  vel_eci : Inport  Port=4
  surface_center : Inport  Port=5
  surface normal : Inport  Port=6
  surface area : Inport  Port=7
  2-norm : Toolbox/vector blocks/2-norm  SystemSampleTime=-1  VariantActivationTime=update diagram  AllowFlexibleInterface=on  Latency=0  AutoFrameSizeCalculation=off
      settings: SourceProductName=SSC flight toolbox
  Add : Sum
  COM : Constant  Value=COM
  Constant : Constant  Value=1/2
  Constant1 : Constant  Value=P_solar
  Constant2 : Constant
  Constant3 : Constant  Value=alpha_acc
  Cross Product : matrix_library/Cross Product
  Cross Product1 : matrix_library/Cross Product
  Dot Product1 : DotProduct  OutDataTypeStr=Inherit: Inherit via internal rule
  Dot Product4 : DotProduct  OutDataTypeStr=Inherit: Inherit via internal rule
  Gain : Gain  Gain=-1
  Gain1 : Gain  Gain=-1
  Nomalize_noDivideByZero : Subsystem
      mask Display: disp('u/||u||')
  Nomalize_noDivideByZero1 : Subsystem
      mask Display: disp('u/||u||')
  Product : Product  Inputs=3
  Product1 : Product  Inputs=4
  Product4 : Product
  Product6 : Product  Inputs=4
  Quaternion Rotation : aerolibutil/Quaternion Rotation
  Quaternion Rotation1 : aerolibutil/Quaternion Rotation
  Square : Math  Operator=square
  Subtract : Sum  Inputs=+-
  Subtract1 : Sum  Inputs=+-
  Switch1 : Switch  Criteria=u2 > Threshold  SaturateOnIntegerOverflow=off  InputSameDT=off
  Switch2 : Switch  Criteria=u2 > Threshold  SaturateOnIntegerOverflow=off  InputSameDT=off
  no sun : Constant  Value=0
  z + area3 : Constant  Value=0
  proj area : Outport
  N_aero_scb : Outport  Port=2
  N_srp_scb : Outport  Port=3
  wires:
  Nomalize_noDivideByZero/1(ehat) -> Add/1, Dot Product4/1  "norm(v)_scb"
  surface area/1 -> Product1/1, Switch2/1  "surface area"
  z + area3/1 -> Switch2/3
  Switch2/1 -> Product4/2
  Product4/1 -> Product6/2, proj area/1
  Dot Product4/1 -> Product4/1, Switch2/2
  rho/1 -> Product6/1
  2-norm/1 -> Square/1
  surface normal/1 -> Dot Product4/2, Product/2, Dot Product1/2  "surface normal"
  Constant/1 -> Product/3
  Product/1 -> Add/2
  Gain/1 -> Product6/4
  Product6/1 -> Cross Product/2
  Cross Product/1 -> N_aero_scb/1
  surface_center/1 -> Subtract/1
  COM/1 -> Subtract/2
  Subtract/1 -> Cross Product1/1, Cross Product/1
  Nomalize_noDivideByZero1/1(ehat) -> Product1/3, Dot Product1/1
  Dot Product1/1 -> Switch1/2, Switch1/1  "sun dot prod"
  Constant1/1 -> Gain1/1
  Gain1/1 -> Product1/2
  Product1/1 -> Cross Product1/2
  Cross Product1/1 -> N_srp_scb/1
  vel_eci/1 -> 2-norm/1, Quaternion Rotation/2
  qECI2scb/1 -> Quaternion Rotation1/1, Quaternion Rotation/1
  Quaternion Rotation/1 -> Nomalize_noDivideByZero/1(e)
  solar_X/1 -> Quaternion Rotation1/2
  Quaternion Rotation1/1 -> Nomalize_noDivideByZero1/1(e)  "sol_pos_scb"
  Add/1 -> Gain/1
  Square/1 -> Product6/3
  Switch1/1 -> Product1/4
  no sun/1 -> Switch1/3
  Constant2/1 -> Subtract1/1
  Constant3/1 -> Subtract1/2
  Subtract1/1 -> Product/1

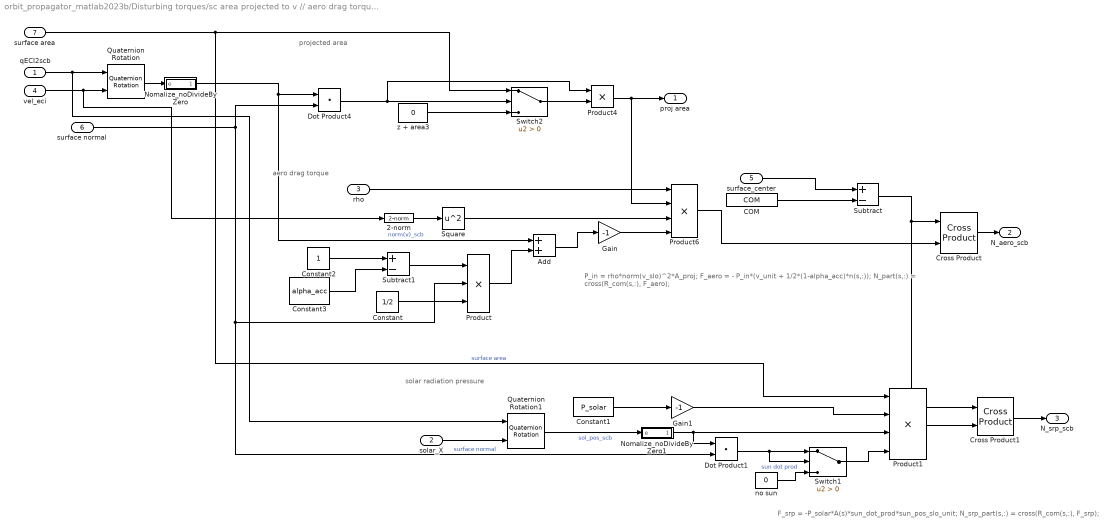
== system orbit_propagator_matlab2023b/Disturbing torques/sc area projected to v // aero drag torque // srp torque/z -2 ==
  note: projected area
  note: aero drag torque
  note: solar radiation pressure
  note: P_in = rho*norm(v_slo)^2*A_proj;
      | F_aero = - P_in*(v_unit + 1/2*(1-alpha_acc)*n(s,:));
      | N_part(s,:) = cross(R_com(s,:), F_aero);
  note: F_srp = -P_solar*A(s)*sun_dot_prod*sun_pos_slo_unit;
      | N_srp_part(s,:) = cross(R_com(s,:), F_srp);
  qECI2scb : Inport
  solar_X : Inport  Port=2
  rho : Inport  Port=3
  vel_eci : Inport  Port=4
  surface_center : Inport  Port=5
  surface normal : Inport  Port=6
  surface area : Inport  Port=7
  2-norm : Toolbox/vector blocks/2-norm  SystemSampleTime=-1  VariantActivationTime=update diagram  AllowFlexibleInterface=on  Latency=0  AutoFrameSizeCalculation=off
      settings: SourceProductName=SSC flight toolbox
  Add : Sum
  COM : Constant  Value=COM
  Constant : Constant  Value=1/2
  Constant1 : Constant  Value=P_solar
  Constant2 : Constant
  Constant3 : Constant  Value=alpha_acc
  Cross Product : matrix_library/Cross Product
  Cross Product1 : matrix_library/Cross Product
  Dot Product1 : DotProduct  OutDataTypeStr=Inherit: Inherit via internal rule
  Dot Product4 : DotProduct  OutDataTypeStr=Inherit: Inherit via internal rule
  Gain : Gain  Gain=-1
  Gain1 : Gain  Gain=-1
  Nomalize_noDivideByZero : Subsystem
      mask Display: disp('u/||u||')
  Nomalize_noDivideByZero1 : Subsystem
      mask Display: disp('u/||u||')
  Product : Product  Inputs=3
  Product1 : Product  Inputs=4
  Product4 : Product
  Product6 : Product  Inputs=4
  Quaternion Rotation : aerolibutil/Quaternion Rotation
  Quaternion Rotation1 : aerolibutil/Quaternion Rotation
  Square : Math  Operator=square
  Subtract : Sum  Inputs=+-
  Subtract1 : Sum  Inputs=+-
  Switch1 : Switch  Criteria=u2 > Threshold  SaturateOnIntegerOverflow=off  InputSameDT=off
  Switch2 : Switch  Criteria=u2 > Threshold  SaturateOnIntegerOverflow=off  InputSameDT=off
  no sun : Constant  Value=0
  z + area3 : Constant  Value=0
  proj area : Outport
  N_aero_scb : Outport  Port=2
  N_srp_scb : Outport  Port=3
  wires:
  Nomalize_noDivideByZero/1(ehat) -> Add/1, Dot Product4/1  "norm(v)_scb"
  surface area/1 -> Product1/1, Switch2/1  "surface area"
  z + area3/1 -> Switch2/3
  Switch2/1 -> Product4/2
  Product4/1 -> Product6/2, proj area/1
  Dot Product4/1 -> Product4/1, Switch2/2
  rho/1 -> Product6/1
  2-norm/1 -> Square/1
  surface normal/1 -> Dot Product4/2, Product/2, Dot Product1/2  "surface normal"
  Constant/1 -> Product/3
  Product/1 -> Add/2
  Gain/1 -> Product6/4
  Product6/1 -> Cross Product/2
  Cross Product/1 -> N_aero_scb/1
  surface_center/1 -> Subtract/1
  COM/1 -> Subtract/2
  Subtract/1 -> Cross Product1/1, Cross Product/1
  Nomalize_noDivideByZero1/1(ehat) -> Product1/3, Dot Product1/1
  Dot Product1/1 -> Switch1/2, Switch1/1  "sun dot prod"
  Constant1/1 -> Gain1/1
  Gain1/1 -> Product1/2
  Product1/1 -> Cross Product1/2
  Cross Product1/1 -> N_srp_scb/1
  vel_eci/1 -> 2-norm/1, Quaternion Rotation/2
  qECI2scb/1 -> Quaternion Rotation1/1, Quaternion Rotation/1
  Quaternion Rotation/1 -> Nomalize_noDivideByZero/1(e)
  solar_X/1 -> Quaternion Rotation1/2
  Quaternion Rotation1/1 -> Nomalize_noDivideByZero1/1(e)  "sol_pos_scb"
  Add/1 -> Gain/1
  Square/1 -> Product6/3
  Switch1/1 -> Product1/4
  no sun/1 -> Switch1/3
  Constant2/1 -> Subtract1/1
  Constant3/1 -> Subtract1/2
  Subtract1/1 -> Product/1

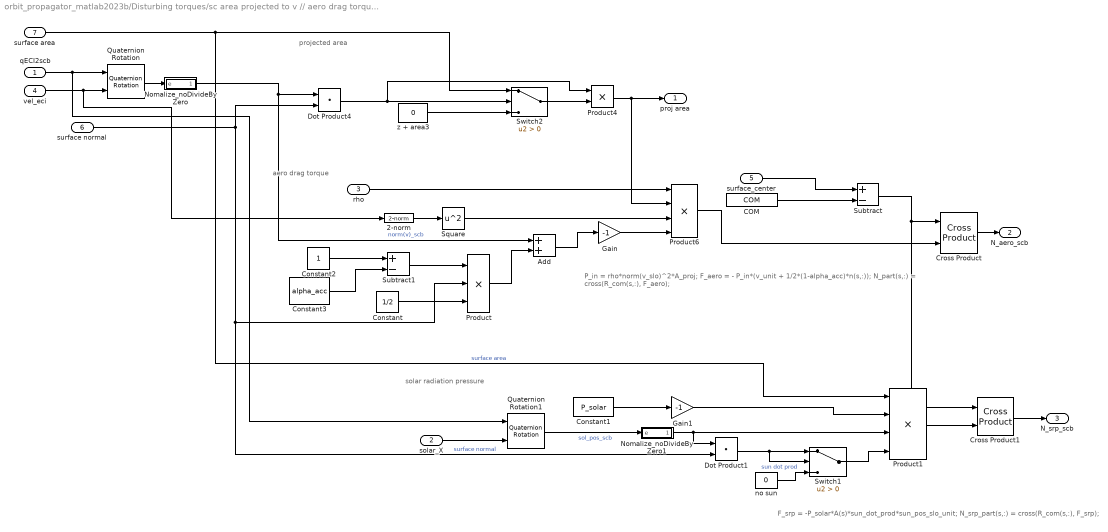
== system orbit_propagator_matlab2023b/Disturbing torques/sc area projected to v // aero drag torque // srp torque/z -3 ==
  note: projected area
  note: aero drag torque
  note: solar radiation pressure
  note: P_in = rho*norm(v_slo)^2*A_proj;
      | F_aero = - P_in*(v_unit + 1/2*(1-alpha_acc)*n(s,:));
      | N_part(s,:) = cross(R_com(s,:), F_aero);
  note: F_srp = -P_solar*A(s)*sun_dot_prod*sun_pos_slo_unit;
      | N_srp_part(s,:) = cross(R_com(s,:), F_srp);
  qECI2scb : Inport
  solar_X : Inport  Port=2
  rho : Inport  Port=3
  vel_eci : Inport  Port=4
  surface_center : Inport  Port=5
  surface normal : Inport  Port=6
  surface area : Inport  Port=7
  2-norm : Toolbox/vector blocks/2-norm  SystemSampleTime=-1  VariantActivationTime=update diagram  AllowFlexibleInterface=on  Latency=0  AutoFrameSizeCalculation=off
      settings: SourceProductName=SSC flight toolbox
  Add : Sum
  COM : Constant  Value=COM
  Constant : Constant  Value=1/2
  Constant1 : Constant  Value=P_solar
  Constant2 : Constant
  Constant3 : Constant  Value=alpha_acc
  Cross Product : matrix_library/Cross Product
  Cross Product1 : matrix_library/Cross Product
  Dot Product1 : DotProduct  OutDataTypeStr=Inherit: Inherit via internal rule
  Dot Product4 : DotProduct  OutDataTypeStr=Inherit: Inherit via internal rule
  Gain : Gain  Gain=-1
  Gain1 : Gain  Gain=-1
  Nomalize_noDivideByZero : Subsystem
      mask Display: disp('u/||u||')
  Nomalize_noDivideByZero1 : Subsystem
      mask Display: disp('u/||u||')
  Product : Product  Inputs=3
  Product1 : Product  Inputs=4
  Product4 : Product
  Product6 : Product  Inputs=4
  Quaternion Rotation : aerolibutil/Quaternion Rotation
  Quaternion Rotation1 : aerolibutil/Quaternion Rotation
  Square : Math  Operator=square
  Subtract : Sum  Inputs=+-
  Subtract1 : Sum  Inputs=+-
  Switch1 : Switch  Criteria=u2 > Threshold  SaturateOnIntegerOverflow=off  InputSameDT=off
  Switch2 : Switch  Criteria=u2 > Threshold  SaturateOnIntegerOverflow=off  InputSameDT=off
  no sun : Constant  Value=0
  z + area3 : Constant  Value=0
  proj area : Outport
  N_aero_scb : Outport  Port=2
  N_srp_scb : Outport  Port=3
  wires:
  Nomalize_noDivideByZero/1(ehat) -> Add/1, Dot Product4/1  "norm(v)_scb"
  surface area/1 -> Product1/1, Switch2/1  "surface area"
  z + area3/1 -> Switch2/3
  Switch2/1 -> Product4/2
  Product4/1 -> Product6/2, proj area/1
  Dot Product4/1 -> Product4/1, Switch2/2
  rho/1 -> Product6/1
  2-norm/1 -> Square/1
  surface normal/1 -> Dot Product4/2, Product/2, Dot Product1/2  "surface normal"
  Constant/1 -> Product/3
  Product/1 -> Add/2
  Gain/1 -> Product6/4
  Product6/1 -> Cross Product/2
  Cross Product/1 -> N_aero_scb/1
  surface_center/1 -> Subtract/1
  COM/1 -> Subtract/2
  Subtract/1 -> Cross Product1/1, Cross Product/1
  Nomalize_noDivideByZero1/1(ehat) -> Product1/3, Dot Product1/1
  Dot Product1/1 -> Switch1/2, Switch1/1  "sun dot prod"
  Constant1/1 -> Gain1/1
  Gain1/1 -> Product1/2
  Product1/1 -> Cross Product1/2
  Cross Product1/1 -> N_srp_scb/1
  vel_eci/1 -> 2-norm/1, Quaternion Rotation/2
  qECI2scb/1 -> Quaternion Rotation1/1, Quaternion Rotation/1
  Quaternion Rotation/1 -> Nomalize_noDivideByZero/1(e)
  solar_X/1 -> Quaternion Rotation1/2
  Quaternion Rotation1/1 -> Nomalize_noDivideByZero1/1(e)  "sol_pos_scb"
  Add/1 -> Gain/1
  Square/1 -> Product6/3
  Switch1/1 -> Product1/4
  no sun/1 -> Switch1/3
  Constant2/1 -> Subtract1/1
  Constant3/1 -> Subtract1/2
  Subtract1/1 -> Product/1

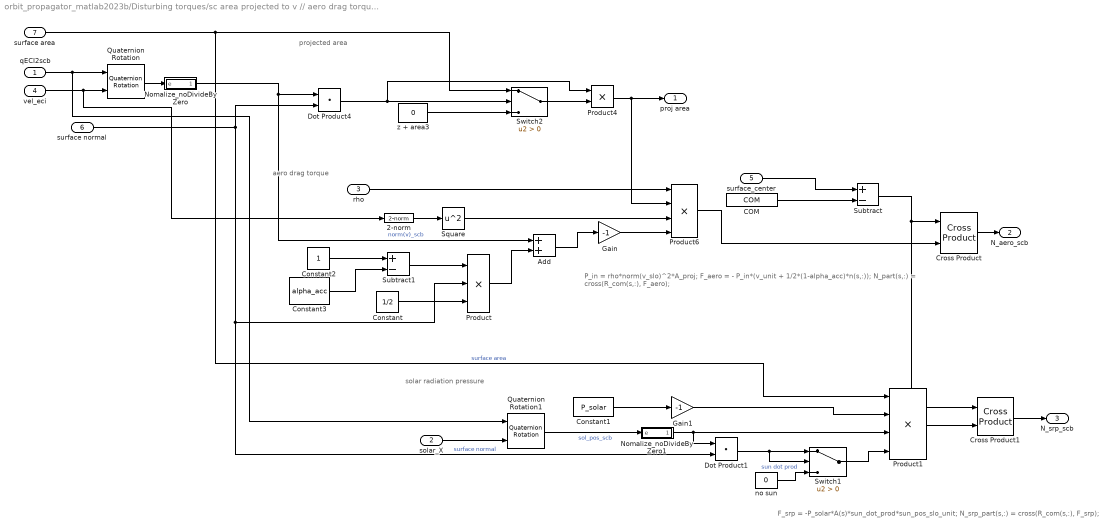
== system orbit_propagator_matlab2023b/Disturbing torques/sc area projected to v // aero drag torque // srp torque/z -4 ==
  note: projected area
  note: aero drag torque
  note: solar radiation pressure
  note: P_in = rho*norm(v_slo)^2*A_proj;
      | F_aero = - P_in*(v_unit + 1/2*(1-alpha_acc)*n(s,:));
      | N_part(s,:) = cross(R_com(s,:), F_aero);
  note: F_srp = -P_solar*A(s)*sun_dot_prod*sun_pos_slo_unit;
      | N_srp_part(s,:) = cross(R_com(s,:), F_srp);
  qECI2scb : Inport
  solar_X : Inport  Port=2
  rho : Inport  Port=3
  vel_eci : Inport  Port=4
  surface_center : Inport  Port=5
  surface normal : Inport  Port=6
  surface area : Inport  Port=7
  2-norm : Toolbox/vector blocks/2-norm  SystemSampleTime=-1  VariantActivationTime=update diagram  AllowFlexibleInterface=on  Latency=0  AutoFrameSizeCalculation=off
      settings: SourceProductName=SSC flight toolbox
  Add : Sum
  COM : Constant  Value=COM
  Constant : Constant  Value=1/2
  Constant1 : Constant  Value=P_solar
  Constant2 : Constant
  Constant3 : Constant  Value=alpha_acc
  Cross Product : matrix_library/Cross Product
  Cross Product1 : matrix_library/Cross Product
  Dot Product1 : DotProduct  OutDataTypeStr=Inherit: Inherit via internal rule
  Dot Product4 : DotProduct  OutDataTypeStr=Inherit: Inherit via internal rule
  Gain : Gain  Gain=-1
  Gain1 : Gain  Gain=-1
  Nomalize_noDivideByZero : Subsystem
      mask Display: disp('u/||u||')
  Nomalize_noDivideByZero1 : Subsystem
      mask Display: disp('u/||u||')
  Product : Product  Inputs=3
  Product1 : Product  Inputs=4
  Product4 : Product
  Product6 : Product  Inputs=4
  Quaternion Rotation : aerolibutil/Quaternion Rotation
  Quaternion Rotation1 : aerolibutil/Quaternion Rotation
  Square : Math  Operator=square
  Subtract : Sum  Inputs=+-
  Subtract1 : Sum  Inputs=+-
  Switch1 : Switch  Criteria=u2 > Threshold  SaturateOnIntegerOverflow=off  InputSameDT=off
  Switch2 : Switch  Criteria=u2 > Threshold  SaturateOnIntegerOverflow=off  InputSameDT=off
  no sun : Constant  Value=0
  z + area3 : Constant  Value=0
  proj area : Outport
  N_aero_scb : Outport  Port=2
  N_srp_scb : Outport  Port=3
  wires:
  Nomalize_noDivideByZero/1(ehat) -> Add/1, Dot Product4/1  "norm(v)_scb"
  surface area/1 -> Product1/1, Switch2/1  "surface area"
  z + area3/1 -> Switch2/3
  Switch2/1 -> Product4/2
  Product4/1 -> Product6/2, proj area/1
  Dot Product4/1 -> Product4/1, Switch2/2
  rho/1 -> Product6/1
  2-norm/1 -> Square/1
  surface normal/1 -> Dot Product4/2, Product/2, Dot Product1/2  "surface normal"
  Constant/1 -> Product/3
  Product/1 -> Add/2
  Gain/1 -> Product6/4
  Product6/1 -> Cross Product/2
  Cross Product/1 -> N_aero_scb/1
  surface_center/1 -> Subtract/1
  COM/1 -> Subtract/2
  Subtract/1 -> Cross Product1/1, Cross Product/1
  Nomalize_noDivideByZero1/1(ehat) -> Product1/3, Dot Product1/1
  Dot Product1/1 -> Switch1/2, Switch1/1  "sun dot prod"
  Constant1/1 -> Gain1/1
  Gain1/1 -> Product1/2
  Product1/1 -> Cross Product1/2
  Cross Product1/1 -> N_srp_scb/1
  vel_eci/1 -> 2-norm/1, Quaternion Rotation/2
  qECI2scb/1 -> Quaternion Rotation1/1, Quaternion Rotation/1
  Quaternion Rotation/1 -> Nomalize_noDivideByZero/1(e)
  solar_X/1 -> Quaternion Rotation1/2
  Quaternion Rotation1/1 -> Nomalize_noDivideByZero1/1(e)  "sol_pos_scb"
  Add/1 -> Gain/1
  Square/1 -> Product6/3
  Switch1/1 -> Product1/4
  no sun/1 -> Switch1/3
  Constant2/1 -> Subtract1/1
  Constant3/1 -> Subtract1/2
  Subtract1/1 -> Product/1

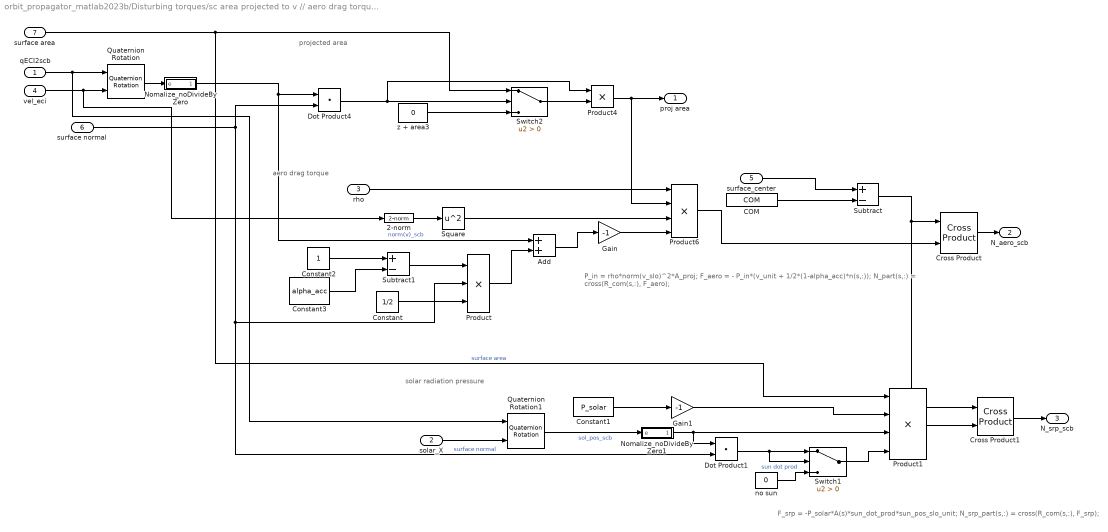
== system orbit_propagator_matlab2023b/Disturbing torques/sc area projected to v // aero drag torque // srp torque/z -5 ==
  note: projected area
  note: aero drag torque
  note: solar radiation pressure
  note: P_in = rho*norm(v_slo)^2*A_proj;
      | F_aero = - P_in*(v_unit + 1/2*(1-alpha_acc)*n(s,:));
      | N_part(s,:) = cross(R_com(s,:), F_aero);
  note: F_srp = -P_solar*A(s)*sun_dot_prod*sun_pos_slo_unit;
      | N_srp_part(s,:) = cross(R_com(s,:), F_srp);
  qECI2scb : Inport
  solar_X : Inport  Port=2
  rho : Inport  Port=3
  vel_eci : Inport  Port=4
  surface_center : Inport  Port=5
  surface normal : Inport  Port=6
  surface area : Inport  Port=7
  2-norm : Toolbox/vector blocks/2-norm  SystemSampleTime=-1  VariantActivationTime=update diagram  AllowFlexibleInterface=on  Latency=0  AutoFrameSizeCalculation=off
      settings: SourceProductName=SSC flight toolbox
  Add : Sum
  COM : Constant  Value=COM
  Constant : Constant  Value=1/2
  Constant1 : Constant  Value=P_solar
  Constant2 : Constant
  Constant3 : Constant  Value=alpha_acc
  Cross Product : matrix_library/Cross Product
  Cross Product1 : matrix_library/Cross Product
  Dot Product1 : DotProduct  OutDataTypeStr=Inherit: Inherit via internal rule
  Dot Product4 : DotProduct  OutDataTypeStr=Inherit: Inherit via internal rule
  Gain : Gain  Gain=-1
  Gain1 : Gain  Gain=-1
  Nomalize_noDivideByZero : Subsystem
      mask Display: disp('u/||u||')
  Nomalize_noDivideByZero1 : Subsystem
      mask Display: disp('u/||u||')
  Product : Product  Inputs=3
  Product1 : Product  Inputs=4
  Product4 : Product
  Product6 : Product  Inputs=4
  Quaternion Rotation : aerolibutil/Quaternion Rotation
  Quaternion Rotation1 : aerolibutil/Quaternion Rotation
  Square : Math  Operator=square
  Subtract : Sum  Inputs=+-
  Subtract1 : Sum  Inputs=+-
  Switch1 : Switch  Criteria=u2 > Threshold  SaturateOnIntegerOverflow=off  InputSameDT=off
  Switch2 : Switch  Criteria=u2 > Threshold  SaturateOnIntegerOverflow=off  InputSameDT=off
  no sun : Constant  Value=0
  z + area3 : Constant  Value=0
  proj area : Outport
  N_aero_scb : Outport  Port=2
  N_srp_scb : Outport  Port=3
  wires:
  Nomalize_noDivideByZero/1(ehat) -> Add/1, Dot Product4/1  "norm(v)_scb"
  surface area/1 -> Product1/1, Switch2/1  "surface area"
  z + area3/1 -> Switch2/3
  Switch2/1 -> Product4/2
  Product4/1 -> Product6/2, proj area/1
  Dot Product4/1 -> Product4/1, Switch2/2
  rho/1 -> Product6/1
  2-norm/1 -> Square/1
  surface normal/1 -> Dot Product4/2, Product/2, Dot Product1/2  "surface normal"
  Constant/1 -> Product/3
  Product/1 -> Add/2
  Gain/1 -> Product6/4
  Product6/1 -> Cross Product/2
  Cross Product/1 -> N_aero_scb/1
  surface_center/1 -> Subtract/1
  COM/1 -> Subtract/2
  Subtract/1 -> Cross Product1/1, Cross Product/1
  Nomalize_noDivideByZero1/1(ehat) -> Product1/3, Dot Product1/1
  Dot Product1/1 -> Switch1/2, Switch1/1  "sun dot prod"
  Constant1/1 -> Gain1/1
  Gain1/1 -> Product1/2
  Product1/1 -> Cross Product1/2
  Cross Product1/1 -> N_srp_scb/1
  vel_eci/1 -> 2-norm/1, Quaternion Rotation/2
  qECI2scb/1 -> Quaternion Rotation1/1, Quaternion Rotation/1
  Quaternion Rotation/1 -> Nomalize_noDivideByZero/1(e)
  solar_X/1 -> Quaternion Rotation1/2
  Quaternion Rotation1/1 -> Nomalize_noDivideByZero1/1(e)  "sol_pos_scb"
  Add/1 -> Gain/1
  Square/1 -> Product6/3
  Switch1/1 -> Product1/4
  no sun/1 -> Switch1/3
  Constant2/1 -> Subtract1/1
  Constant3/1 -> Subtract1/2
  Subtract1/1 -> Product/1
